simulink model "gab"  (R2021a)
settings: Solver=VariableStepAuto  StartTime=0.0  StopTime=10.0  RelTol=1e-3
libraries: simulink x1
settings Model: Creator=DaniSan  LastModifiedBy=DaniSan

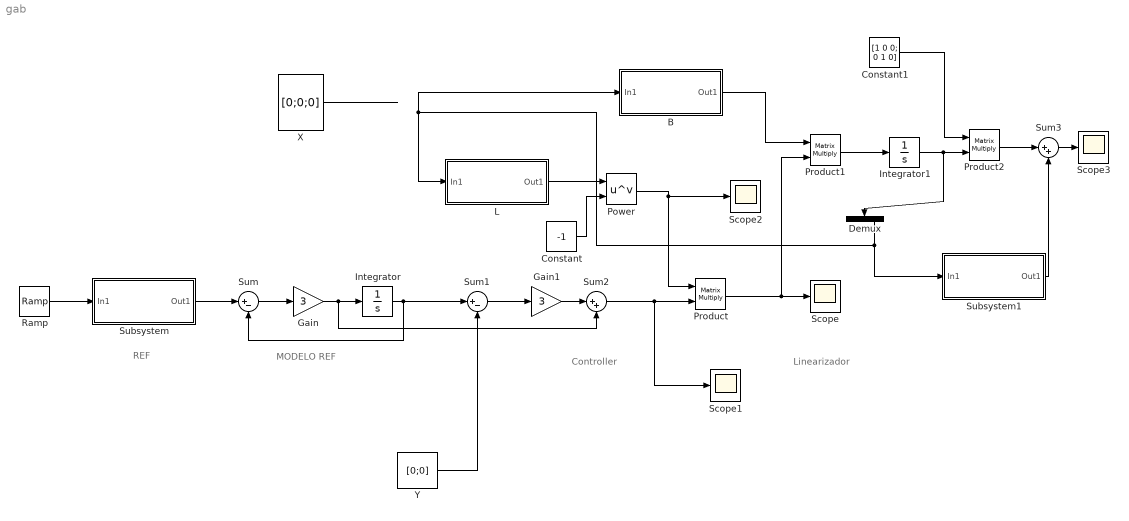
== system gab ==
  note: Linearizador
  note: Controller
  note: MODELO REF
  note: REF
  B : Subsystem
  Constant : Constant  Value=-1
  Constant1 : Constant  Value=[1 0 0; 0 1 0]  VectorParams1D=off
  Demux : Demux  Outputs=3
  Gain : Gain  Gain=3
  Gain1 : Gain  Gain=3
  Integrator : Integrator
  Integrator1 : Integrator
  L : Subsystem
  Power : Math  Operator=pow  SaturateOnIntegerOverflow=on
  Product : Product  Multiplication=Matrix(*)
  Product1 : Product  Multiplication=Matrix(*)
  Product2 : Product  Multiplication=Matrix(*)
  Ramp : simulink/Sources/Ramp  slope=1  start=0  InitialOutput=0
  Scope{,1..3} (4 alike) : Scope
  Subsystem : Subsystem
  Subsystem1 : Subsystem
  Sum : Sum  Inputs=|+-
  Sum1 : Sum  Inputs=|+-
  Sum2 : Sum  Inputs=|++
  Sum3 : Sum  Inputs=|++
  X : Constant  Value=[0;0;0]  VectorParams1D=off
  Y : Constant  Value=[0;0]  VectorParams1D=off
  wires:
  Ramp/1 -> Subsystem/1(In1)
  Subsystem/1(Out1) -> Sum/1
  Gain/1 -> Sum2/2, Integrator/1
  Sum/1 -> Gain/1
  Integrator/1 -> Sum1/1, Sum/2
  Y/1 -> Sum1/2
  Sum1/1 -> Gain1/1
  Gain1/1 -> Sum2/1
  Sum2/1 -> Scope1/1, Product/2
  X/1 -> ?
  Demux/3 -> Subsystem1/1(In1), L/1(In1), B/1(In1)
  Constant/1 -> Power/2
  L/1(Out1) -> Power/1
  Power/1 -> Product/1, Scope2/1
  Product/1 -> Product1/2, Scope/1
  B/1(Out1) -> Product1/1
  Integrator1/1 -> Product2/2, Demux/1
  Product1/1 -> Integrator1/1
  Constant1/1 -> Product2/1
  Product2/1 -> Sum3/1
  Subsystem1/1(Out1) -> Sum3/2
  Sum3/1 -> Scope3/1

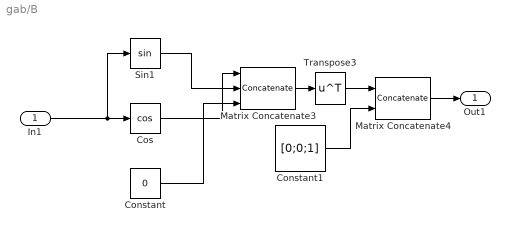
== system gab/B ==
  In1 : Inport
  Constant : Constant  Value=0
  Constant1 : Constant  Value=[0;0;1]  VectorParams1D=off
  Cos : Trigonometry  Operator=cos
  Matrix Concatenate3 : Concatenate  NumInputs=3  Mode=Multidimensional array  ConcatenateDimension=2
  Matrix Concatenate4 : Concatenate  Mode=Multidimensional array  ConcatenateDimension=2
  Sin1 : Trigonometry
  Transpose3 : Math  Operator=transpose  SaturateOnIntegerOverflow=on
  Out1 : Outport
  wires:
  In1/1 -> Sin1/1, Cos/1
  Sin1/1 -> Matrix Concatenate3/2
  Cos/1 -> Matrix Concatenate3/1
  Constant/1 -> Matrix Concatenate3/3
  Matrix Concatenate3/1 -> Transpose3/1
  Constant1/1 -> Matrix Concatenate4/2
  Transpose3/1 -> Matrix Concatenate4/1
  Matrix Concatenate4/1 -> Out1/1

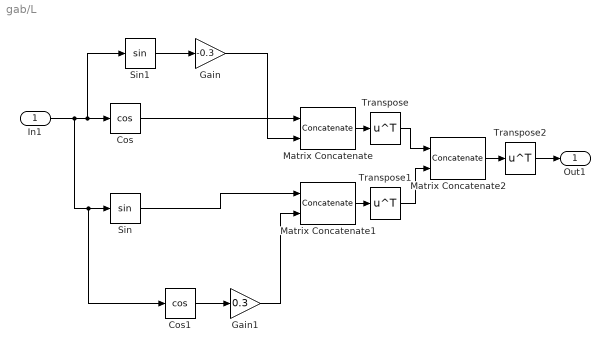
== system gab/L ==
  In1 : Inport
  Cos : Trigonometry  Operator=cos
  Cos1 : Trigonometry  Operator=cos
  Gain : Gain  Gain=-0.3
  Gain1 : Gain  Gain=0.3
  Matrix Concatenate : Concatenate  Mode=Multidimensional array  ConcatenateDimension=2
  Matrix Concatenate1 : Concatenate  Mode=Multidimensional array  ConcatenateDimension=2
  Matrix Concatenate2 : Concatenate  Mode=Multidimensional array  ConcatenateDimension=2
  Sin : Trigonometry
  Sin1 : Trigonometry
  Transpose : Math  Operator=transpose  SaturateOnIntegerOverflow=on
  Transpose1 : Math  Operator=transpose  SaturateOnIntegerOverflow=on
  Transpose2 : Math  Operator=transpose  SaturateOnIntegerOverflow=on
  Out1 : Outport
  wires:
  In1/1 -> Cos1/1, Sin/1, Sin1/1, Cos/1
  Sin1/1 -> Gain/1
  Gain/1 -> Matrix Concatenate/2
  Cos/1 -> Matrix Concatenate/1
  Cos1/1 -> Gain1/1
  Gain1/1 -> Matrix Concatenate1/2
  Sin/1 -> Matrix Concatenate1/1
  Matrix Concatenate/1 -> Transpose/1
  Matrix Concatenate1/1 -> Transpose1/1
  Transpose/1 -> Matrix Concatenate2/1
  Transpose1/1 -> Matrix Concatenate2/2
  Matrix Concatenate2/1 -> Transpose2/1
  Transpose2/1 -> Out1/1

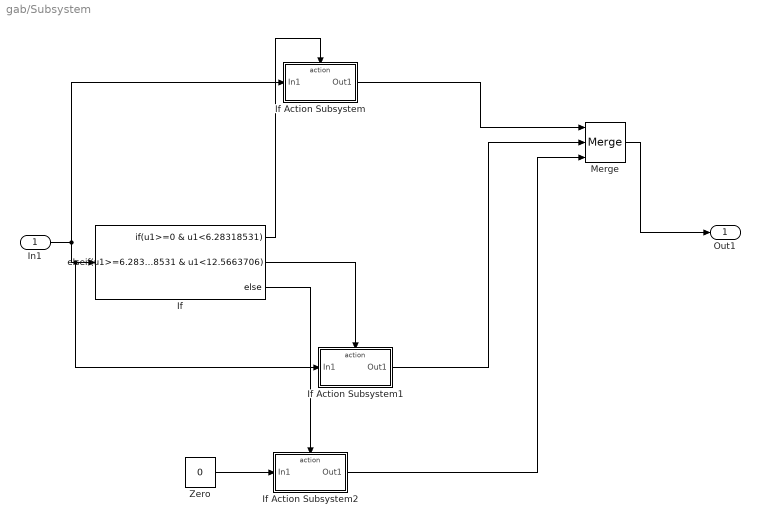
== system gab/Subsystem ==
  In1 : Inport
  If : If  IfExpression=u1>=0 & u1<6.28318531  ElseIfExpressions=u1>=6.28318531 & u1<12.5663706
  If Action Subsystem : Subsystem  TreatAsAtomicUnit=on
  If Action Subsystem1 : Subsystem  TreatAsAtomicUnit=on
  If Action Subsystem2 : Subsystem  TreatAsAtomicUnit=on
  Merge : Merge  Inputs=3
  Zero : Constant  Value=0  OutDataTypeStr=Inherit: Inherit via back propagation
  Out1 : Outport
  wires:
  In1/1 -> If Action Subsystem/1(In1), If Action Subsystem1/1(In1), If/1
  Merge/1 -> Out1/1
  If/1 -> If Action Subsystem/Action
  If Action Subsystem/1(Out1) -> Merge/1
  If/2 -> If Action Subsystem1/Action
  If/3 -> If Action Subsystem2/Action
  Zero/1 -> If Action Subsystem2/1(In1)
  If Action Subsystem1/1(Out1) -> Merge/2
  If Action Subsystem2/1(Out1) -> Merge/3

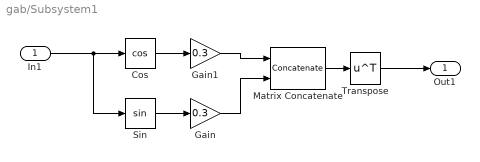
== system gab/Subsystem1 ==
  In1 : Inport
  Cos : Trigonometry  Operator=cos
  Gain : Gain  Gain=0.3
  Gain1 : Gain  Gain=0.3
  Matrix Concatenate : Concatenate  Mode=Multidimensional array  ConcatenateDimension=2
  Sin : Trigonometry
  Transpose : Math  Operator=transpose  SaturateOnIntegerOverflow=on
  Out1 : Outport
  wires:
  In1/1 -> Sin/1, Cos/1
  Cos/1 -> Gain1/1
  Sin/1 -> Gain/1
  Gain1/1 -> Matrix Concatenate/1
  Gain/1 -> Matrix Concatenate/2
  Matrix Concatenate/1 -> Transpose/1
  Transpose/1 -> Out1/1

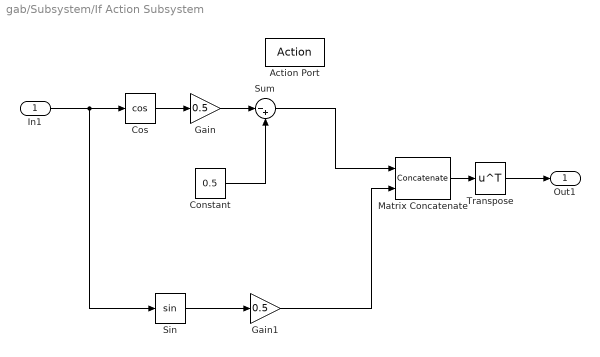
== system gab/Subsystem/If Action Subsystem ==
  In1 : Inport
  Action Port : ActionPort  ActionPortLabel=if(u1>=0 & u1<6.28318531)
  Constant : Constant  Value=0.5
  Cos : Trigonometry  Operator=cos
  Gain : Gain  Gain=0.5
  Gain1 : Gain  Gain=0.5
  Matrix Concatenate : Concatenate  Mode=Multidimensional array  ConcatenateDimension=2
  Sin : Trigonometry
  Sum : Sum  Inputs=|-+
  Transpose : Math  Operator=transpose  SaturateOnIntegerOverflow=on
  Out1 : Outport
  wires:
  In1/1 -> Sin/1, Cos/1
  Constant/1 -> Sum/2
  Gain/1 -> Sum/1
  Cos/1 -> Gain/1
  Sum/1 -> Matrix Concatenate/1
  Sin/1 -> Gain1/1
  Gain1/1 -> Matrix Concatenate/2
  Matrix Concatenate/1 -> Transpose/1
  Transpose/1 -> Out1/1

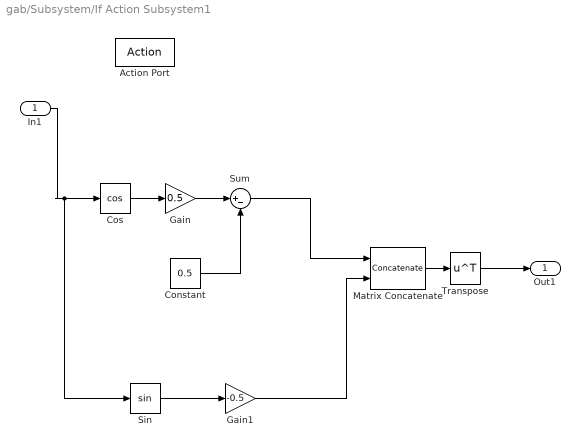
== system gab/Subsystem/If Action Subsystem1 ==
  In1 : Inport
  Action Port : ActionPort  ActionPortLabel=elseif(u1>=6.28318531 & u1<12.5663706)
  Constant : Constant  Value=0.5
  Cos : Trigonometry  Operator=cos
  Gain : Gain  Gain=0.5
  Gain1 : Gain  Gain=-0.5
  Matrix Concatenate : Concatenate  Mode=Multidimensional array  ConcatenateDimension=2
  Sin : Trigonometry
  Sum : Sum  Inputs=|+-
  Transpose : Math  Operator=transpose  SaturateOnIntegerOverflow=on
  Out1 : Outport
  wires:
  Sin/1 -> Gain1/1
  Transpose/1 -> Out1/1
  Matrix Concatenate/1 -> Transpose/1
  Sum/1 -> Matrix Concatenate/1
  Gain/1 -> Sum/1
  Cos/1 -> Gain/1
  Gain1/1 -> Matrix Concatenate/2
  Constant/1 -> Sum/2
  In1/1 -> Sin/1, Cos/1

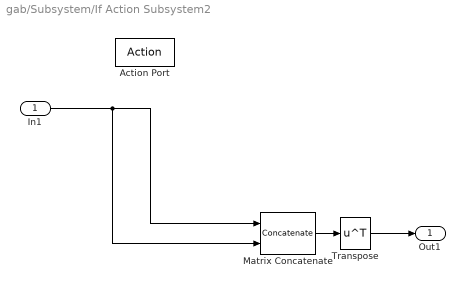
== system gab/Subsystem/If Action Subsystem2 ==
  In1 : Inport
  Action Port : ActionPort  ActionPortLabel=else
  Matrix Concatenate : Concatenate  Mode=Multidimensional array  ConcatenateDimension=2
  Transpose : Math  Operator=transpose  SaturateOnIntegerOverflow=on
  Out1 : Outport
  wires:
  In1/1 -> Matrix Concatenate/2, Matrix Concatenate/1
  Matrix Concatenate/1 -> Transpose/1
  Transpose/1 -> Out1/1
